simulink model "enable_DTI"  (R2016a)
settings: Solver=VariableStepAuto  StartTime=0.0  StopTime=10.0  RelTol=1e-3
undefined symbols (not defined in the file): DiscIntNeverNeededParam
settings Model: Creator=hamza  LastModifiedBy=hamza

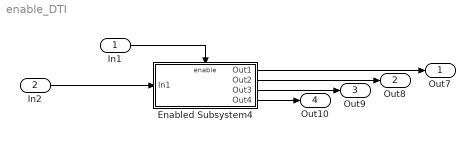
== system enable_DTI ==
  In1 : Inport  OutDataTypeStr=boolean
  In2 : Inport  Port=2  OutDataTypeStr=double
  Enabled Subsystem4 : Subsystem  TreatAsAtomicUnit=on
  Out7 : Outport
  Out8 : Outport  Port=2
  Out9 : Outport  Port=3
  Out10 : Outport  Port=4
  wires:
  In2/1 -> Enabled Subsystem4/1(In1)
  Enabled Subsystem4/1(Out1) -> Out7/1
  In1/1 -> Enabled Subsystem4/Enable
  Enabled Subsystem4/2(Out2) -> Out8/1
  Enabled Subsystem4/3(Out3) -> Out9/1
  Enabled Subsystem4/4(Out4) -> Out10/1

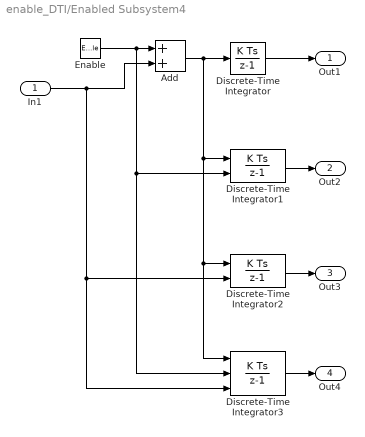
== system enable_DTI/Enabled Subsystem4 ==
  In1 : Inport
  Enable : EnablePort  StatesWhenEnabling=reset  ShowOutputPort=on
  Add : Sum
  Discrete-Time Integrator : DiscreteIntegrator  InitialConditionSetting=State (most efficient)  ICPrevOutput=DiscIntNeverNeededParam  ICPrevScaledInput=DiscIntNeverNeededParam
  Discrete-Time Integrator1 : DiscreteIntegrator  ExternalReset=falling  InitialConditionSetting=State (most efficient)  ICPrevOutput=DiscIntNeverNeededParam  ICPrevScaledInput=DiscIntNeverNeededParam
  Discrete-Time Integrator2 : DiscreteIntegrator  InitialConditionSource=external  InitialConditionSetting=State (most efficient)  ICPrevOutput=DiscIntNeverNeededParam  ICPrevScaledInput=DiscIntNeverNeededParam
  Discrete-Time Integrator3 : DiscreteIntegrator  ExternalReset=level  InitialConditionSource=external  InitialConditionSetting=State (most efficient)  ICPrevOutput=DiscIntNeverNeededParam  ICPrevScaledInput=DiscIntNeverNeededParam
  Out1 : Outport
  Out2 : Outport  Port=2
  Out3 : Outport  Port=3
  Out4 : Outport  Port=4
  wires:
  Enable/1 -> Discrete-Time Integrator3/2, Discrete-Time Integrator1/2, Add/1
  In1/1 -> Discrete-Time Integrator3/3, Discrete-Time Integrator2/2, Add/2
  Add/1 -> Discrete-Time Integrator3/1, Discrete-Time Integrator2/1, Discrete-Time Integrator1/1, Discrete-Time Integrator/1
  Discrete-Time Integrator/1 -> Out1/1
  Discrete-Time Integrator1/1 -> Out2/1
  Discrete-Time Integrator2/1 -> Out3/1
  Discrete-Time Integrator3/1 -> Out4/1
